simulink model "q2_2"  (R2026a)
settings: Solver=VariableStepAuto  StopTime=0.5
undefined symbols (not defined in the file): DiscIntNeverNeededParam
libraries: dspfdesign x1
settings Model: Creator=steve  LastModifiedBy=steve

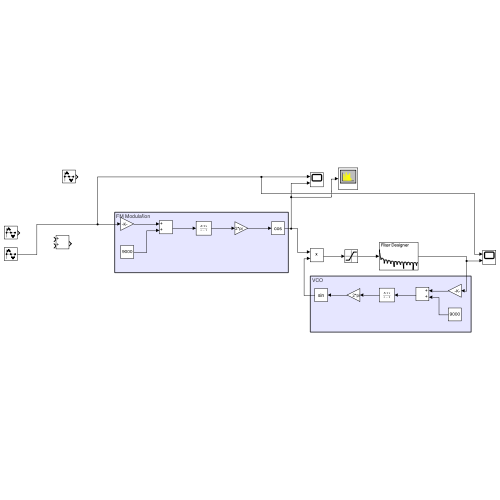
[thumbnail: Simulink's stored preview of the top-level diagram]
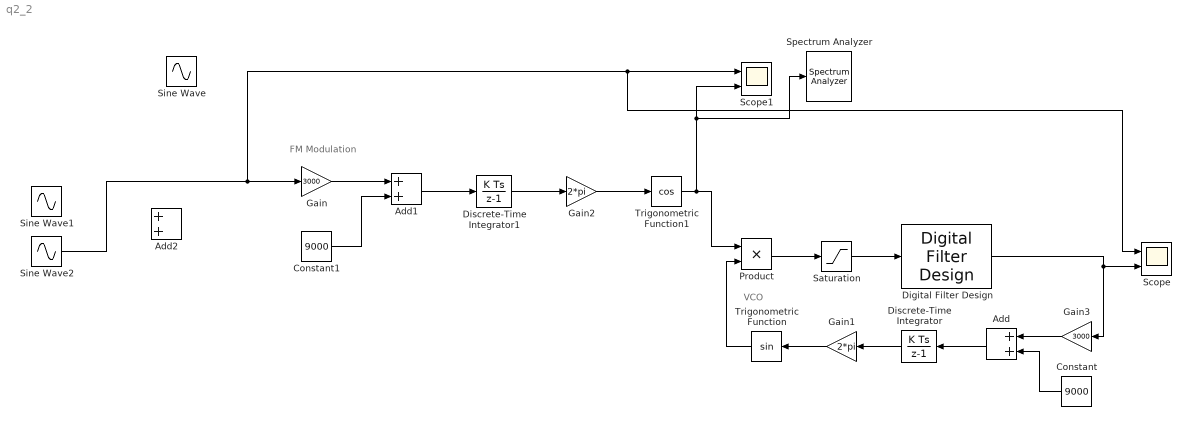
== system q2_2 ==
  note: VCO
  note: FM Modulation
  Add : Sum
  Add1 : Sum
  Add2 : Sum
  Constant : Constant  Value=9000
  Constant1 : Constant  Value=9000
  Digital Filter Design : dspfdesign/Digital Filter Design  mwdsp_browser_bugfix_var=off
  Discrete-Time Integrator : DiscreteIntegrator  SampleTime=-1  ICPrevOutput=DiscIntNeverNeededParam  ICPrevScaledInput=DiscIntNeverNeededParam
  Discrete-Time Integrator1 : DiscreteIntegrator  SampleTime=1e-6  ICPrevOutput=DiscIntNeverNeededParam  ICPrevScaledInput=DiscIntNeverNeededParam
  Gain : Gain  Gain=3000
  Gain1 : Gain  Gain=2*pi
  Gain2 : Gain  Gain=2*pi
  Gain3 : Gain  Gain=3000
  Product : Product
  Saturation : Saturate
  Scope : Scope  NumInputPorts=2
  Scope1 : Scope  NumInputPorts=2
      settings: ActiveDisplayYMinimum=-1.25  ActiveDisplayYMaximum=1.25
  Sine Wave : Sin  SineType=Sample based  Samples=1000  SampleTime=1e-6
  Sine Wave1 : Sin  SineType=Sample based  Samples=1000  SampleTime=1e-6
  Sine Wave2 : Sin  SineType=Sample based  Samples=500  SampleTime=1e-6
  Spectrum Analyzer : SpectrumAnalyzer  WindowPosition=[357.000000,34.000000,800.000000,500.000000,]  ScopeFrameLocation=window  WindowInvariantSamplesPerUpdate=on  YLimits=[-255.1109 48.0268]
  Trigonometric Function : Trigonometry
  Trigonometric Function1 : Trigonometry  Operator=cos
  wires:
  Gain/1 -> Add1/1
  Constant1/1 -> Add1/2
  Add1/1 -> Discrete-Time Integrator1/1
  Discrete-Time Integrator1/1 -> Gain2/1
  Gain2/1 -> Trigonometric Function1/1
  Product/1 -> Saturation/1
  Saturation/1 -> Digital Filter Design/1
  Digital Filter Design/1 -> Gain3/1, Scope/2
  Constant/1 -> Add/2
  Add/1 -> Discrete-Time Integrator/1
  Gain1/1 -> Trigonometric Function/1
  Discrete-Time Integrator/1 -> Gain1/1
  Trigonometric Function/1 -> Product/2
  Gain3/1 -> Add/1
  Trigonometric Function1/1 -> Product/1, Spectrum Analyzer/1, Scope1/2
  Sine Wave2/1 -> Scope/1, Scope1/1, Gain/1
